simulink model "simu3"  (R2022a)
settings: Solver=VariableStepAuto  StartTime=0.0  StopTime=10.0  RelTol=1e-3
values from neighbouring files (symbols this model uses):
  x0 = 0    [lista08.m]
settings Model: Creator=marcone.faria  LastModifiedBy=marcone.faria

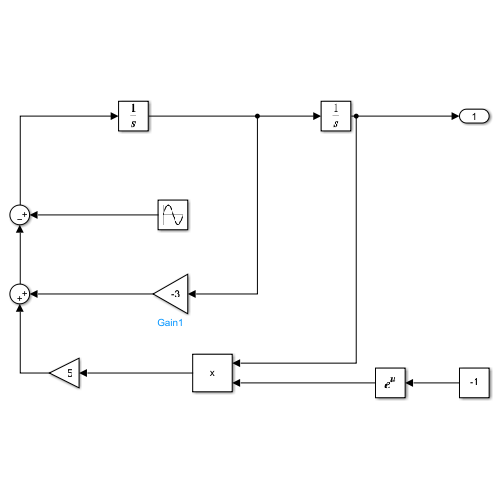
[thumbnail: Simulink's stored preview of the top-level diagram]
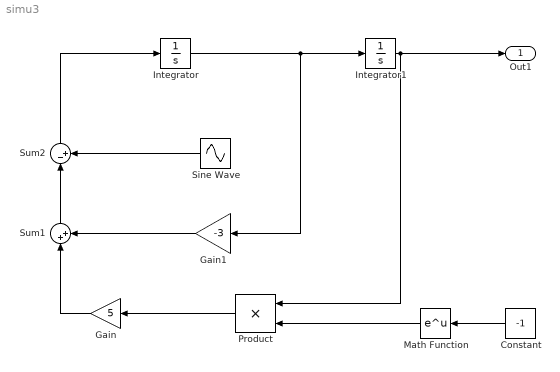
== system simu3 ==
  Constant : Constant  Value=-1
  Gain : Gain  Gain=5
  Gain1 : Gain  Gain=-3
  Integrator : Integrator  InitialCondition=x0
  Integrator1 : Integrator  InitialCondition=x0
  Math Function : Math
  Product : Product
  Sine Wave : Sin  Amplitude=8  Frequency=5  SampleTime=0
  Sum1 : Sum  Inputs=|++
  Sum2 : Sum  Inputs=|-+
  Out1 : Outport
  wires:
  Integrator/1 -> Gain1/1, Integrator1/1
  Integrator1/1 -> Out1/1, Product/1
  Sine Wave/1 -> Sum2/2
  Sum2/1 -> Integrator/1
  Sum1/1 -> Sum2/1
  Gain1/1 -> Sum1/2
  Gain/1 -> Sum1/1
  Product/1 -> Gain/1
  Math Function/1 -> Product/2
  Constant/1 -> Math Function/1
